simulink model "ExampleMotive_control_communication_2015a"  (R2015a)
settings: Solver=ode1  StartTime=0.0  StopTime=inf  FixedStep=0.2  RelTol=1e-3
settings Model: ExtModeTrigDuration=5000  Creator=adm-drone  LastModifiedBy=jitesh_esb201
settings SolverCC: PositivePriorityOrder=on
settings DebuggingCC: UnderspecifiedInitializationDetection=Classic  MergeDetectMultiDrivingBlocksExec=none  SolverPrmCheckMsg=warning  StateNameClashWarn=warning
settings RTWCC: SystemTargetFile=quarc_win64.tlc  TemplateMakefile=quarc_default_tmf  Description=QUARC Win64 Target
settings STFCustomTargetCC: TargetLibSuffix=.lib  TargetPreCompLibLocation=C:\PROGRA~3\QUARC\lib\2013a\win64\release  GenerateSampleERTMain=off  GeneratePreprocessorConditionals=Disable all  CombineOutputUpdateFcns=on  ERTCustomFileBanners=off  SupportNonInlinedSFcns=on  SupportVariableSizeSignals=off  MATLABClassNameForMDSCustomization=Simulink.SoftwareTarget.GRTCustomization  CPPClassGenCompliant=on  SystemTargetFile=quarc_win64.tlc
settings GRTTargetCC: TargetPreCompLibLocation=C:\PROGRA~3\QUARC\lib\2013a\win64\release  ParMdlRefBuildCompliant=off  CompOptLevelCompliant=off  ConcurrentExecutionCompliant=off  MatFileLogging=off  ExtMode=on  ExtModeMexFile=quarc_comm

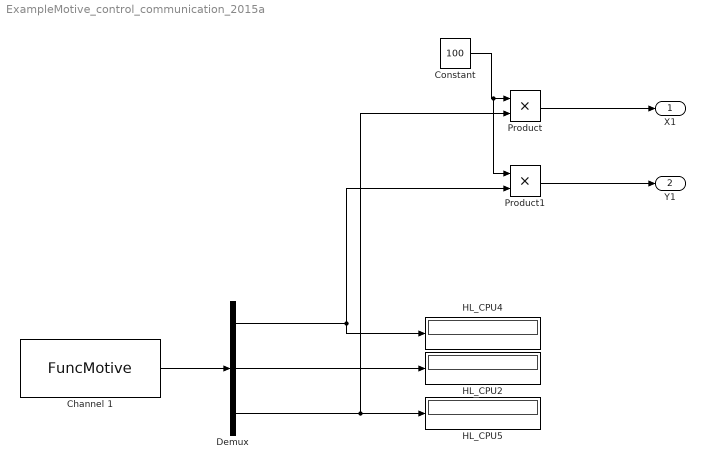
== system ExampleMotive_control_communication_2015a ==
  Channel 1 : M-S-Function  FunctionName=FuncMotive  Parameters=1
  Constant : Constant  Value=100
  Demux : Demux  Outputs=3
  HL_CPU2 : Display
  HL_CPU4 : Display
  HL_CPU5 : Display
  Product : Product
  Product1 : Product
  X1 : Outport
  Y1 : Outport  Port=2
  wires:
  Channel 1/1 -> Demux/1
  Demux/1 -> HL_CPU4/1, Product1/2
  Demux/2 -> HL_CPU2/1
  Demux/3 -> Product/2, HL_CPU5/1
  Constant/1 -> Product1/1, Product/1
  Product/1 -> X1/1
  Product1/1 -> Y1/1
